simulink model "speedgoat_test_SN5659_R2021b"  (R2021b)
settings: Solver=FixedStepDiscrete  StartTime=0.0  StopTime=inf  RelTol=1e-3
PreLoadFcn:
  | Ts_IO107 = 0.001;
  | Ts_IO107 = 0.001;
  | Ts_IO133 = 0.001
  | 
  | Ts_IO204 = 0.001;
  | 
  | 
  | Ts_IO503 = 0.01;
  | 
  | ts_IO612 = 1e-3;
  | Ts_IO682 = 0.005;
  | Ts_IO941 = 0.01;
InitFcn:
  | Ts_IO107 = 0.001;
  | Ts_IO107 = 0.001;
  | Ts_IO133 = 0.001
  | 
  | Ts_IO204 = 0.001;
  | 
  | 
  | Ts_IO503 = 0.01;
  | 
  | ts_IO612 = 1e-3;
  | Ts_IO682 = 0.005;
  | Ts_IO941 = 0.01;
StopFcn:
  | if isfile(['sdi_view_',bdroot,'.mldatx'])
  |  Simulink.sdi.clearPreferences();
  |  Simulink.sdi.view();
  |  pause(3);
  |  Simulink.sdi.loadView(['sdi_view_',bdroot,]);
  | end
undefined symbols (not defined in the file): C, IO682, standard
libraries: speedgoatlib_IO682 x161, simulink x49, slrealtimeseriallib x16, canmsglib x12, speedgoatlib_serial x9, speedgoatlib_IO612 x9, speedgoatlib_IO133 x5, speedgoatlib_IO107 x4, speedgoatlib_IO204 x3, speedgoatlib_IO421 x3, speedgoatlib_PIL x1
(part 2 of 4)

== system speedgoat_test_SN5659_R2021b/IO682/Decode Channel 12 ==
  In1 : Inport
  Decode 1 : speedgoatlib_IO682/Decode v2   parMode=Standard  parLabel=100  parDataType=[1]  parResolution=[1024]  parSyncMask=hex2dec('0x0')  parSyncValue=hex2dec('0x0')  parCustomDataType=Raw  parDataLSB=9  parDataMSB=31  parBitPosition=[9, 31]  parScaleBNR=1  parExponent=8  parMantissa=14  parTimeTags=off  parHoldLastVal=on  parStatus=off
      settings: SourceProductName=Simulink Real-Time: Speedgoat I/O Blockset
  Decode 2 : speedgoatlib_IO682/Decode v2   parMode=Standard  parLabel=101  parDataType=[2]  parResolution=[.1]  parSyncMask=hex2dec('0x0')  parSyncValue=hex2dec('0x0')  parCustomDataType=Raw  parDataLSB=9  parDataMSB=31  parBitPosition=[9, 31]  parScaleBNR=1  parExponent=8  parMantissa=14  parTimeTags=off  parHoldLastVal=on  parStatus=off
      settings: SourceProductName=Simulink Real-Time: Speedgoat I/O Blockset
  Decode 3 : speedgoatlib_IO682/Decode v2   parMode=Standard  parLabel=102  parDataType=[1]  parResolution=[65536]  parSyncMask=hex2dec('0x0')  parSyncValue=hex2dec('0x0')  parCustomDataType=Raw  parDataLSB=9  parDataMSB=31  parBitPosition=[9, 31]  parScaleBNR=1  parExponent=8  parMantissa=14  parTimeTags=off  parHoldLastVal=on  parStatus=off
      settings: SourceProductName=Simulink Real-Time: Speedgoat I/O Blockset
  Decode 4 : speedgoatlib_IO682/Decode v2   parMode=Standard  parLabel=103  parDataType=[1]  parResolution=[1024]  parSyncMask=hex2dec('0x0')  parSyncValue=hex2dec('0x0')  parCustomDataType=Raw  parDataLSB=9  parDataMSB=31  parBitPosition=[9, 31]  parScaleBNR=1  parExponent=8  parMantissa=14  parTimeTags=off  parHoldLastVal=on  parStatus=off
      settings: SourceProductName=Simulink Real-Time: Speedgoat I/O Blockset
  Mux : Mux
  Out1 : Outport
  wires:
  Decode 1/1 -> Mux/1
  Decode 2/1 -> Mux/2
  Decode 4/1 -> Mux/4
  Decode 3/1 -> Mux/3
  Mux/1 -> Out1/1
  In1/1 -> Decode 4/1, Decode 3/1, Decode 2/1, Decode 1/1

== system speedgoat_test_SN5659_R2021b/IO682/Decode Channel 13 ==
  note: Because of the limited number of bits
      | that are encoded and sent by ARINC,
      | these values may differ from values
      | on the input side.
  In1 : Inport
  Decode 1 : speedgoatlib_IO682/Decode v2   parMode=Standard  parLabel=100  parDataType=[1]  parResolution=[1024]  parSyncMask=hex2dec('0x0')  parSyncValue=hex2dec('0x0')  parCustomDataType=Raw  parDataLSB=9  parDataMSB=31  parBitPosition=[9, 31]  parScaleBNR=1  parExponent=8  parMantissa=14  parTimeTags=off  parHoldLastVal=on  parStatus=off
      settings: SourceProductName=Simulink Real-Time: Speedgoat I/O Blockset
  Decode 3 : speedgoatlib_IO682/Decode v2   parMode=Standard  parLabel=102  parDataType=[1]  parResolution=[65536]  parSyncMask=hex2dec('0x0')  parSyncValue=hex2dec('0x0')  parCustomDataType=Raw  parDataLSB=9  parDataMSB=31  parBitPosition=[9, 31]  parScaleBNR=1  parExponent=8  parMantissa=14  parTimeTags=off  parHoldLastVal=on  parStatus=off
      settings: SourceProductName=Simulink Real-Time: Speedgoat I/O Blockset
  Decode 4 : speedgoatlib_IO682/Decode v2   parMode=Standard  parLabel=103  parDataType=[1]  parResolution=[1024]  parSyncMask=hex2dec('0x0')  parSyncValue=hex2dec('0x0')  parCustomDataType=Raw  parDataLSB=9  parDataMSB=31  parBitPosition=[9, 31]  parScaleBNR=1  parExponent=8  parMantissa=14  parTimeTags=off  parHoldLastVal=on  parStatus=off
      settings: SourceProductName=Simulink Real-Time: Speedgoat I/O Blockset
  Decode 5 : speedgoatlib_IO682/Decode v2   parMode=Standard  parLabel=101  parDataType=[2]  parResolution=[.1]  parSyncMask=hex2dec('0x0')  parSyncValue=hex2dec('0x0')  parCustomDataType=Raw  parDataLSB=9  parDataMSB=31  parBitPosition=[9, 31]  parScaleBNR=1  parExponent=8  parMantissa=14  parTimeTags=off  parHoldLastVal=on  parStatus=off
      settings: SourceProductName=Simulink Real-Time: Speedgoat I/O Blockset
  Mux : Mux
  Out1 : Outport
  wires:
  In1/1 -> Decode 3/1, Decode 4/1, Decode 5/1, Decode 1/1
  Mux/1 -> Out1/1
  Decode 5/1 -> Mux/2
  Decode 1/1 -> Mux/1
  Decode 3/1 -> Mux/3
  Decode 4/1 -> Mux/4

== system speedgoat_test_SN5659_R2021b/IO682/Decode Channel 14 ==
  In1 : Inport
  Decode 1 : speedgoatlib_IO682/Decode v2   parMode=Standard  parLabel=100  parDataType=[1]  parResolution=[1024]  parSyncMask=hex2dec('0x0')  parSyncValue=hex2dec('0x0')  parCustomDataType=Raw  parDataLSB=9  parDataMSB=31  parBitPosition=[9, 31]  parScaleBNR=1  parExponent=8  parMantissa=14  parTimeTags=off  parHoldLastVal=on  parStatus=off
      settings: SourceProductName=Simulink Real-Time: Speedgoat I/O Blockset
  Decode 2 : speedgoatlib_IO682/Decode v2   parMode=Standard  parLabel=101  parDataType=[2]  parResolution=[.1]  parSyncMask=hex2dec('0x0')  parSyncValue=hex2dec('0x0')  parCustomDataType=Raw  parDataLSB=9  parDataMSB=31  parBitPosition=[9, 31]  parScaleBNR=1  parExponent=8  parMantissa=14  parTimeTags=off  parHoldLastVal=on  parStatus=off
      settings: SourceProductName=Simulink Real-Time: Speedgoat I/O Blockset
  Decode 3 : speedgoatlib_IO682/Decode v2   parMode=Standard  parLabel=102  parDataType=[1]  parResolution=[65536]  parSyncMask=hex2dec('0x0')  parSyncValue=hex2dec('0x0')  parCustomDataType=Raw  parDataLSB=9  parDataMSB=31  parBitPosition=[9, 31]  parScaleBNR=1  parExponent=8  parMantissa=14  parTimeTags=off  parHoldLastVal=on  parStatus=off
      settings: SourceProductName=Simulink Real-Time: Speedgoat I/O Blockset
  Decode 4 : speedgoatlib_IO682/Decode v2   parMode=Standard  parLabel=103  parDataType=[1]  parResolution=[1024]  parSyncMask=hex2dec('0x0')  parSyncValue=hex2dec('0x0')  parCustomDataType=Raw  parDataLSB=9  parDataMSB=31  parBitPosition=[9, 31]  parScaleBNR=1  parExponent=8  parMantissa=14  parTimeTags=off  parHoldLastVal=on  parStatus=off
      settings: SourceProductName=Simulink Real-Time: Speedgoat I/O Blockset
  Mux : Mux
  Out1 : Outport
  wires:
  Decode 1/1 -> Mux/1
  In1/1 -> Decode 4/1, Decode 3/1, Decode 2/1, Decode 1/1
  Mux/1 -> Out1/1
  Decode 4/1 -> Mux/4
  Decode 3/1 -> Mux/3
  Decode 2/1 -> Mux/2

== system speedgoat_test_SN5659_R2021b/IO682/Decode Channel 15 ==
  In1 : Inport
  Decode 1 : speedgoatlib_IO682/Decode v2   parMode=Standard  parLabel=100  parDataType=[1]  parResolution=[1024]  parSyncMask=hex2dec('0x0')  parSyncValue=hex2dec('0x0')  parCustomDataType=Raw  parDataLSB=9  parDataMSB=31  parBitPosition=[9, 31]  parScaleBNR=1  parExponent=8  parMantissa=14  parTimeTags=off  parHoldLastVal=on  parStatus=off
      settings: SourceProductName=Simulink Real-Time: Speedgoat I/O Blockset
  Decode 2 : speedgoatlib_IO682/Decode v2   parMode=Standard  parLabel=101  parDataType=[2]  parResolution=[.1]  parSyncMask=hex2dec('0x0')  parSyncValue=hex2dec('0x0')  parCustomDataType=Raw  parDataLSB=9  parDataMSB=31  parBitPosition=[9, 31]  parScaleBNR=1  parExponent=8  parMantissa=14  parTimeTags=off  parHoldLastVal=on  parStatus=off
      settings: SourceProductName=Simulink Real-Time: Speedgoat I/O Blockset
  Decode 3 : speedgoatlib_IO682/Decode v2   parMode=Standard  parLabel=102  parDataType=[1]  parResolution=[65536]  parSyncMask=hex2dec('0x0')  parSyncValue=hex2dec('0x0')  parCustomDataType=Raw  parDataLSB=9  parDataMSB=31  parBitPosition=[9, 31]  parScaleBNR=1  parExponent=8  parMantissa=14  parTimeTags=off  parHoldLastVal=on  parStatus=off
      settings: SourceProductName=Simulink Real-Time: Speedgoat I/O Blockset
  Decode 4 : speedgoatlib_IO682/Decode v2   parMode=Standard  parLabel=103  parDataType=[1]  parResolution=[1024]  parSyncMask=hex2dec('0x0')  parSyncValue=hex2dec('0x0')  parCustomDataType=Raw  parDataLSB=9  parDataMSB=31  parBitPosition=[9, 31]  parScaleBNR=1  parExponent=8  parMantissa=14  parTimeTags=off  parHoldLastVal=on  parStatus=off
      settings: SourceProductName=Simulink Real-Time: Speedgoat I/O Blockset
  Mux : Mux
  Out1 : Outport
  wires:
  Decode 1/1 -> Mux/1
  Decode 2/1 -> Mux/2
  Decode 4/1 -> Mux/4
  Decode 3/1 -> Mux/3
  Mux/1 -> Out1/1
  In1/1 -> Decode 4/1, Decode 3/1, Decode 2/1, Decode 1/1

== system speedgoat_test_SN5659_R2021b/IO682/Decode Channel 16 ==
  In1 : Inport
  Decode 1 : speedgoatlib_IO682/Decode v2   parMode=Standard  parLabel=100  parDataType=[1]  parResolution=[1024]  parSyncMask=hex2dec('0x0')  parSyncValue=hex2dec('0x0')  parCustomDataType=Raw  parDataLSB=9  parDataMSB=31  parBitPosition=[9, 31]  parScaleBNR=1  parExponent=8  parMantissa=14  parTimeTags=off  parHoldLastVal=on  parStatus=off
      settings: SourceProductName=Simulink Real-Time: Speedgoat I/O Blockset
  Decode 2 : speedgoatlib_IO682/Decode v2   parMode=Standard  parLabel=101  parDataType=[2]  parResolution=[.1]  parSyncMask=hex2dec('0x0')  parSyncValue=hex2dec('0x0')  parCustomDataType=Raw  parDataLSB=9  parDataMSB=31  parBitPosition=[9, 31]  parScaleBNR=1  parExponent=8  parMantissa=14  parTimeTags=off  parHoldLastVal=on  parStatus=off
      settings: SourceProductName=Simulink Real-Time: Speedgoat I/O Blockset
  Decode 3 : speedgoatlib_IO682/Decode v2   parMode=Standard  parLabel=102  parDataType=[1]  parResolution=[65536]  parSyncMask=hex2dec('0x0')  parSyncValue=hex2dec('0x0')  parCustomDataType=Raw  parDataLSB=9  parDataMSB=31  parBitPosition=[9, 31]  parScaleBNR=1  parExponent=8  parMantissa=14  parTimeTags=off  parHoldLastVal=on  parStatus=off
      settings: SourceProductName=Simulink Real-Time: Speedgoat I/O Blockset
  Decode 4 : speedgoatlib_IO682/Decode v2   parMode=Standard  parLabel=103  parDataType=[1]  parResolution=[1024]  parSyncMask=hex2dec('0x0')  parSyncValue=hex2dec('0x0')  parCustomDataType=Raw  parDataLSB=9  parDataMSB=31  parBitPosition=[9, 31]  parScaleBNR=1  parExponent=8  parMantissa=14  parTimeTags=off  parHoldLastVal=on  parStatus=off
      settings: SourceProductName=Simulink Real-Time: Speedgoat I/O Blockset
  Mux : Mux
  Out1 : Outport
  wires:
  Decode 1/1 -> Mux/1
  Decode 2/1 -> Mux/2
  Decode 4/1 -> Mux/4
  Decode 3/1 -> Mux/3
  Mux/1 -> Out1/1
  In1/1 -> Decode 4/1, Decode 3/1, Decode 2/1, Decode 1/1

== system speedgoat_test_SN5659_R2021b/IO682/Decode Channel 2 ==
  In1 : Inport
  Decode 1 : speedgoatlib_IO682/Decode v2   parMode=Standard  parLabel=100  parDataType=[1]  parResolution=[1024]  parSyncMask=hex2dec('0x0')  parSyncValue=hex2dec('0x0')  parCustomDataType=Raw  parDataLSB=9  parDataMSB=31  parBitPosition=[9, 31]  parScaleBNR=1  parExponent=8  parMantissa=14  parTimeTags=off  parHoldLastVal=on  parStatus=off
      settings: SourceProductName=Simulink Real-Time: Speedgoat I/O Blockset
  Decode 2 : speedgoatlib_IO682/Decode v2   parMode=Standard  parLabel=101  parDataType=[2]  parResolution=[.1]  parSyncMask=hex2dec('0x0')  parSyncValue=hex2dec('0x0')  parCustomDataType=Raw  parDataLSB=9  parDataMSB=31  parBitPosition=[9, 31]  parScaleBNR=1  parExponent=8  parMantissa=14  parTimeTags=off  parHoldLastVal=on  parStatus=off
      settings: SourceProductName=Simulink Real-Time: Speedgoat I/O Blockset
  Decode 3 : speedgoatlib_IO682/Decode v2   parMode=Standard  parLabel=102  parDataType=[1]  parResolution=[65536]  parSyncMask=hex2dec('0x0')  parSyncValue=hex2dec('0x0')  parCustomDataType=Raw  parDataLSB=9  parDataMSB=31  parBitPosition=[9, 31]  parScaleBNR=1  parExponent=8  parMantissa=14  parTimeTags=off  parHoldLastVal=on  parStatus=off
      settings: SourceProductName=Simulink Real-Time: Speedgoat I/O Blockset
  Decode 4 : speedgoatlib_IO682/Decode v2   parMode=Standard  parLabel=103  parDataType=[1]  parResolution=[1024]  parSyncMask=hex2dec('0x0')  parSyncValue=hex2dec('0x0')  parCustomDataType=Raw  parDataLSB=9  parDataMSB=31  parBitPosition=[9, 31]  parScaleBNR=1  parExponent=8  parMantissa=14  parTimeTags=off  parHoldLastVal=on  parStatus=off
      settings: SourceProductName=Simulink Real-Time: Speedgoat I/O Blockset
  Mux : Mux
  Out1 : Outport
  wires:
  Decode 1/1 -> Mux/1
  In1/1 -> Decode 4/1, Decode 3/1, Decode 2/1, Decode 1/1
  Mux/1 -> Out1/1
  Decode 4/1 -> Mux/4
  Decode 3/1 -> Mux/3
  Decode 2/1 -> Mux/2

== system speedgoat_test_SN5659_R2021b/IO682/Decode Channel 3 ==
  In1 : Inport
  Decode 1 : speedgoatlib_IO682/Decode v2   parMode=Standard  parLabel=100  parDataType=[1]  parResolution=[1024]  parSyncMask=hex2dec('0x0')  parSyncValue=hex2dec('0x0')  parCustomDataType=Raw  parDataLSB=9  parDataMSB=31  parBitPosition=[9, 31]  parScaleBNR=1  parExponent=8  parMantissa=14  parTimeTags=off  parHoldLastVal=on  parStatus=off
      settings: SourceProductName=Simulink Real-Time: Speedgoat I/O Blockset
  Decode 2 : speedgoatlib_IO682/Decode v2   parMode=Standard  parLabel=101  parDataType=[2]  parResolution=[.1]  parSyncMask=hex2dec('0x0')  parSyncValue=hex2dec('0x0')  parCustomDataType=Raw  parDataLSB=9  parDataMSB=31  parBitPosition=[9, 31]  parScaleBNR=1  parExponent=8  parMantissa=14  parTimeTags=off  parHoldLastVal=on  parStatus=off
      settings: SourceProductName=Simulink Real-Time: Speedgoat I/O Blockset
  Decode 3 : speedgoatlib_IO682/Decode v2   parMode=Standard  parLabel=102  parDataType=[1]  parResolution=[65536]  parSyncMask=hex2dec('0x0')  parSyncValue=hex2dec('0x0')  parCustomDataType=Raw  parDataLSB=9  parDataMSB=31  parBitPosition=[9, 31]  parScaleBNR=1  parExponent=8  parMantissa=14  parTimeTags=off  parHoldLastVal=on  parStatus=off
      settings: SourceProductName=Simulink Real-Time: Speedgoat I/O Blockset
  Decode 4 : speedgoatlib_IO682/Decode v2   parMode=Standard  parLabel=103  parDataType=[1]  parResolution=[1024]  parSyncMask=hex2dec('0x0')  parSyncValue=hex2dec('0x0')  parCustomDataType=Raw  parDataLSB=9  parDataMSB=31  parBitPosition=[9, 31]  parScaleBNR=1  parExponent=8  parMantissa=14  parTimeTags=off  parHoldLastVal=on  parStatus=off
      settings: SourceProductName=Simulink Real-Time: Speedgoat I/O Blockset
  Mux : Mux
  Out1 : Outport
  wires:
  Decode 1/1 -> Mux/1
  Decode 2/1 -> Mux/2
  Decode 4/1 -> Mux/4
  Decode 3/1 -> Mux/3
  Mux/1 -> Out1/1
  In1/1 -> Decode 4/1, Decode 3/1, Decode 2/1, Decode 1/1

== system speedgoat_test_SN5659_R2021b/IO682/Decode Channel 4 ==
  In1 : Inport
  Decode 1 : speedgoatlib_IO682/Decode v2   parMode=Standard  parLabel=100  parDataType=[1]  parResolution=[1024]  parSyncMask=hex2dec('0x0')  parSyncValue=hex2dec('0x0')  parCustomDataType=Raw  parDataLSB=9  parDataMSB=31  parBitPosition=[9, 31]  parScaleBNR=1  parExponent=8  parMantissa=14  parTimeTags=off  parHoldLastVal=on  parStatus=off
      settings: SourceProductName=Simulink Real-Time: Speedgoat I/O Blockset
  Decode 2 : speedgoatlib_IO682/Decode v2   parMode=Standard  parLabel=101  parDataType=[2]  parResolution=[.1]  parSyncMask=hex2dec('0x0')  parSyncValue=hex2dec('0x0')  parCustomDataType=Raw  parDataLSB=9  parDataMSB=31  parBitPosition=[9, 31]  parScaleBNR=1  parExponent=8  parMantissa=14  parTimeTags=off  parHoldLastVal=on  parStatus=off
      settings: SourceProductName=Simulink Real-Time: Speedgoat I/O Blockset
  Decode 3 : speedgoatlib_IO682/Decode v2   parMode=Standard  parLabel=102  parDataType=[1]  parResolution=[65536]  parSyncMask=hex2dec('0x0')  parSyncValue=hex2dec('0x0')  parCustomDataType=Raw  parDataLSB=9  parDataMSB=31  parBitPosition=[9, 31]  parScaleBNR=1  parExponent=8  parMantissa=14  parTimeTags=off  parHoldLastVal=on  parStatus=off
      settings: SourceProductName=Simulink Real-Time: Speedgoat I/O Blockset
  Decode 4 : speedgoatlib_IO682/Decode v2   parMode=Standard  parLabel=103  parDataType=[1]  parResolution=[1024]  parSyncMask=hex2dec('0x0')  parSyncValue=hex2dec('0x0')  parCustomDataType=Raw  parDataLSB=9  parDataMSB=31  parBitPosition=[9, 31]  parScaleBNR=1  parExponent=8  parMantissa=14  parTimeTags=off  parHoldLastVal=on  parStatus=off
      settings: SourceProductName=Simulink Real-Time: Speedgoat I/O Blockset
  Mux : Mux
  Out1 : Outport
  wires:
  Decode 1/1 -> Mux/1
  Decode 2/1 -> Mux/2
  Decode 4/1 -> Mux/4
  Decode 3/1 -> Mux/3
  Mux/1 -> Out1/1
  In1/1 -> Decode 4/1, Decode 3/1, Decode 2/1, Decode 1/1

== system speedgoat_test_SN5659_R2021b/IO682/Decode Channel 5 ==
  note: Because of the limited number of bits
      | that are encoded and sent by ARINC,
      | these values may differ from values
      | on the input side.
  In1 : Inport
  Decode 1 : speedgoatlib_IO682/Decode v2   parMode=Standard  parLabel=100  parDataType=[1]  parResolution=[1024]  parSyncMask=hex2dec('0x0')  parSyncValue=hex2dec('0x0')  parCustomDataType=Raw  parDataLSB=9  parDataMSB=31  parBitPosition=[9, 31]  parScaleBNR=1  parExponent=8  parMantissa=14  parTimeTags=off  parHoldLastVal=on  parStatus=off
      settings: SourceProductName=Simulink Real-Time: Speedgoat I/O Blockset
  Decode 3 : speedgoatlib_IO682/Decode v2   parMode=Standard  parLabel=102  parDataType=[1]  parResolution=[65536]  parSyncMask=hex2dec('0x0')  parSyncValue=hex2dec('0x0')  parCustomDataType=Raw  parDataLSB=9  parDataMSB=31  parBitPosition=[9, 31]  parScaleBNR=1  parExponent=8  parMantissa=14  parTimeTags=off  parHoldLastVal=on  parStatus=off
      settings: SourceProductName=Simulink Real-Time: Speedgoat I/O Blockset
  Decode 4 : speedgoatlib_IO682/Decode v2   parMode=Standard  parLabel=103  parDataType=[1]  parResolution=[1024]  parSyncMask=hex2dec('0x0')  parSyncValue=hex2dec('0x0')  parCustomDataType=Raw  parDataLSB=9  parDataMSB=31  parBitPosition=[9, 31]  parScaleBNR=1  parExponent=8  parMantissa=14  parTimeTags=off  parHoldLastVal=on  parStatus=off
      settings: SourceProductName=Simulink Real-Time: Speedgoat I/O Blockset
  Decode 5 : speedgoatlib_IO682/Decode v2   parMode=Standard  parLabel=101  parDataType=[2]  parResolution=[.1]  parSyncMask=hex2dec('0x0')  parSyncValue=hex2dec('0x0')  parCustomDataType=Raw  parDataLSB=9  parDataMSB=31  parBitPosition=[9, 31]  parScaleBNR=1  parExponent=8  parMantissa=14  parTimeTags=off  parHoldLastVal=on  parStatus=off
      settings: SourceProductName=Simulink Real-Time: Speedgoat I/O Blockset
  Mux : Mux
  Out1 : Outport
  wires:
  In1/1 -> Decode 3/1, Decode 4/1, Decode 5/1, Decode 1/1
  Mux/1 -> Out1/1
  Decode 5/1 -> Mux/2
  Decode 1/1 -> Mux/1
  Decode 3/1 -> Mux/3
  Decode 4/1 -> Mux/4

== system speedgoat_test_SN5659_R2021b/IO682/Decode Channel 6 ==
  In1 : Inport
  Decode 1 : speedgoatlib_IO682/Decode v2   parMode=Standard  parLabel=100  parDataType=[1]  parResolution=[1024]  parSyncMask=hex2dec('0x0')  parSyncValue=hex2dec('0x0')  parCustomDataType=Raw  parDataLSB=9  parDataMSB=31  parBitPosition=[9, 31]  parScaleBNR=1  parExponent=8  parMantissa=14  parTimeTags=off  parHoldLastVal=on  parStatus=off
      settings: SourceProductName=Simulink Real-Time: Speedgoat I/O Blockset
  Decode 2 : speedgoatlib_IO682/Decode v2   parMode=Standard  parLabel=101  parDataType=[2]  parResolution=[.1]  parSyncMask=hex2dec('0x0')  parSyncValue=hex2dec('0x0')  parCustomDataType=Raw  parDataLSB=9  parDataMSB=31  parBitPosition=[9, 31]  parScaleBNR=1  parExponent=8  parMantissa=14  parTimeTags=off  parHoldLastVal=on  parStatus=off
      settings: SourceProductName=Simulink Real-Time: Speedgoat I/O Blockset
  Decode 3 : speedgoatlib_IO682/Decode v2   parMode=Standard  parLabel=102  parDataType=[1]  parResolution=[65536]  parSyncMask=hex2dec('0x0')  parSyncValue=hex2dec('0x0')  parCustomDataType=Raw  parDataLSB=9  parDataMSB=31  parBitPosition=[9, 31]  parScaleBNR=1  parExponent=8  parMantissa=14  parTimeTags=off  parHoldLastVal=on  parStatus=off
      settings: SourceProductName=Simulink Real-Time: Speedgoat I/O Blockset
  Decode 4 : speedgoatlib_IO682/Decode v2   parMode=Standard  parLabel=103  parDataType=[1]  parResolution=[1024]  parSyncMask=hex2dec('0x0')  parSyncValue=hex2dec('0x0')  parCustomDataType=Raw  parDataLSB=9  parDataMSB=31  parBitPosition=[9, 31]  parScaleBNR=1  parExponent=8  parMantissa=14  parTimeTags=off  parHoldLastVal=on  parStatus=off
      settings: SourceProductName=Simulink Real-Time: Speedgoat I/O Blockset
  Mux : Mux
  Out1 : Outport
  wires:
  Decode 1/1 -> Mux/1
  In1/1 -> Decode 4/1, Decode 3/1, Decode 2/1, Decode 1/1
  Mux/1 -> Out1/1
  Decode 4/1 -> Mux/4
  Decode 3/1 -> Mux/3
  Decode 2/1 -> Mux/2

== system speedgoat_test_SN5659_R2021b/IO682/Decode Channel 7 ==
  In1 : Inport
  Decode 1 : speedgoatlib_IO682/Decode v2   parMode=Standard  parLabel=100  parDataType=[1]  parResolution=[1024]  parSyncMask=hex2dec('0x0')  parSyncValue=hex2dec('0x0')  parCustomDataType=Raw  parDataLSB=9  parDataMSB=31  parBitPosition=[9, 31]  parScaleBNR=1  parExponent=8  parMantissa=14  parTimeTags=off  parHoldLastVal=on  parStatus=off
      settings: SourceProductName=Simulink Real-Time: Speedgoat I/O Blockset
  Decode 2 : speedgoatlib_IO682/Decode v2   parMode=Standard  parLabel=101  parDataType=[2]  parResolution=[.1]  parSyncMask=hex2dec('0x0')  parSyncValue=hex2dec('0x0')  parCustomDataType=Raw  parDataLSB=9  parDataMSB=31  parBitPosition=[9, 31]  parScaleBNR=1  parExponent=8  parMantissa=14  parTimeTags=off  parHoldLastVal=on  parStatus=off
      settings: SourceProductName=Simulink Real-Time: Speedgoat I/O Blockset
  Decode 3 : speedgoatlib_IO682/Decode v2   parMode=Standard  parLabel=102  parDataType=[1]  parResolution=[65536]  parSyncMask=hex2dec('0x0')  parSyncValue=hex2dec('0x0')  parCustomDataType=Raw  parDataLSB=9  parDataMSB=31  parBitPosition=[9, 31]  parScaleBNR=1  parExponent=8  parMantissa=14  parTimeTags=off  parHoldLastVal=on  parStatus=off
      settings: SourceProductName=Simulink Real-Time: Speedgoat I/O Blockset
  Decode 4 : speedgoatlib_IO682/Decode v2   parMode=Standard  parLabel=103  parDataType=[1]  parResolution=[1024]  parSyncMask=hex2dec('0x0')  parSyncValue=hex2dec('0x0')  parCustomDataType=Raw  parDataLSB=9  parDataMSB=31  parBitPosition=[9, 31]  parScaleBNR=1  parExponent=8  parMantissa=14  parTimeTags=off  parHoldLastVal=on  parStatus=off
      settings: SourceProductName=Simulink Real-Time: Speedgoat I/O Blockset
  Mux : Mux
  Out1 : Outport
  wires:
  Decode 1/1 -> Mux/1
  Decode 2/1 -> Mux/2
  Decode 4/1 -> Mux/4
  Decode 3/1 -> Mux/3
  Mux/1 -> Out1/1
  In1/1 -> Decode 4/1, Decode 3/1, Decode 2/1, Decode 1/1

== system speedgoat_test_SN5659_R2021b/IO682/Decode Channel 8 ==
  In1 : Inport
  Decode 1 : speedgoatlib_IO682/Decode v2   parMode=Standard  parLabel=100  parDataType=[1]  parResolution=[1024]  parSyncMask=hex2dec('0x0')  parSyncValue=hex2dec('0x0')  parCustomDataType=Raw  parDataLSB=9  parDataMSB=31  parBitPosition=[9, 31]  parScaleBNR=1  parExponent=8  parMantissa=14  parTimeTags=off  parHoldLastVal=on  parStatus=off
      settings: SourceProductName=Simulink Real-Time: Speedgoat I/O Blockset
  Decode 2 : speedgoatlib_IO682/Decode v2   parMode=Standard  parLabel=101  parDataType=[2]  parResolution=[.1]  parSyncMask=hex2dec('0x0')  parSyncValue=hex2dec('0x0')  parCustomDataType=Raw  parDataLSB=9  parDataMSB=31  parBitPosition=[9, 31]  parScaleBNR=1  parExponent=8  parMantissa=14  parTimeTags=off  parHoldLastVal=on  parStatus=off
      settings: SourceProductName=Simulink Real-Time: Speedgoat I/O Blockset
  Decode 3 : speedgoatlib_IO682/Decode v2   parMode=Standard  parLabel=102  parDataType=[1]  parResolution=[65536]  parSyncMask=hex2dec('0x0')  parSyncValue=hex2dec('0x0')  parCustomDataType=Raw  parDataLSB=9  parDataMSB=31  parBitPosition=[9, 31]  parScaleBNR=1  parExponent=8  parMantissa=14  parTimeTags=off  parHoldLastVal=on  parStatus=off
      settings: SourceProductName=Simulink Real-Time: Speedgoat I/O Blockset
  Decode 4 : speedgoatlib_IO682/Decode v2   parMode=Standard  parLabel=103  parDataType=[1]  parResolution=[1024]  parSyncMask=hex2dec('0x0')  parSyncValue=hex2dec('0x0')  parCustomDataType=Raw  parDataLSB=9  parDataMSB=31  parBitPosition=[9, 31]  parScaleBNR=1  parExponent=8  parMantissa=14  parTimeTags=off  parHoldLastVal=on  parStatus=off
      settings: SourceProductName=Simulink Real-Time: Speedgoat I/O Blockset
  Mux : Mux
  Out1 : Outport
  wires:
  Decode 1/1 -> Mux/1
  Decode 2/1 -> Mux/2
  Decode 4/1 -> Mux/4
  Decode 3/1 -> Mux/3
  Mux/1 -> Out1/1
  In1/1 -> Decode 4/1, Decode 3/1, Decode 2/1, Decode 1/1

== system speedgoat_test_SN5659_R2021b/IO682/Decode Channel 9 ==
  note: Because of the limited number of bits
      | that are encoded and sent by ARINC,
      | these values may differ from values
      | on the input side.
  In1 : Inport
  Decode 1 : speedgoatlib_IO682/Decode v2   parMode=Standard  parLabel=100  parDataType=[1]  parResolution=[1024]  parSyncMask=hex2dec('0x0')  parSyncValue=hex2dec('0x0')  parCustomDataType=Raw  parDataLSB=9  parDataMSB=31  parBitPosition=[9, 31]  parScaleBNR=1  parExponent=8  parMantissa=14  parTimeTags=off  parHoldLastVal=on  parStatus=off
      settings: SourceProductName=Simulink Real-Time: Speedgoat I/O Blockset
  Decode 3 : speedgoatlib_IO682/Decode v2   parMode=Standard  parLabel=102  parDataType=[1]  parResolution=[65536]  parSyncMask=hex2dec('0x0')  parSyncValue=hex2dec('0x0')  parCustomDataType=Raw  parDataLSB=9  parDataMSB=31  parBitPosition=[9, 31]  parScaleBNR=1  parExponent=8  parMantissa=14  parTimeTags=off  parHoldLastVal=on  parStatus=off
      settings: SourceProductName=Simulink Real-Time: Speedgoat I/O Blockset
  Decode 4 : speedgoatlib_IO682/Decode v2   parMode=Standard  parLabel=103  parDataType=[1]  parResolution=[1024]  parSyncMask=hex2dec('0x0')  parSyncValue=hex2dec('0x0')  parCustomDataType=Raw  parDataLSB=9  parDataMSB=31  parBitPosition=[9, 31]  parScaleBNR=1  parExponent=8  parMantissa=14  parTimeTags=off  parHoldLastVal=on  parStatus=off
      settings: SourceProductName=Simulink Real-Time: Speedgoat I/O Blockset
  Decode 5 : speedgoatlib_IO682/Decode v2   parMode=Standard  parLabel=101  parDataType=[2]  parResolution=[.1]  parSyncMask=hex2dec('0x0')  parSyncValue=hex2dec('0x0')  parCustomDataType=Raw  parDataLSB=9  parDataMSB=31  parBitPosition=[9, 31]  parScaleBNR=1  parExponent=8  parMantissa=14  parTimeTags=off  parHoldLastVal=on  parStatus=off
      settings: SourceProductName=Simulink Real-Time: Speedgoat I/O Blockset
  Mux : Mux
  Out1 : Outport
  wires:
  In1/1 -> Decode 3/1, Decode 4/1, Decode 5/1, Decode 1/1
  Mux/1 -> Out1/1
  Decode 5/1 -> Mux/2
  Decode 1/1 -> Mux/1
  Decode 3/1 -> Mux/3
  Decode 4/1 -> Mux/4

== system speedgoat_test_SN5659_R2021b/IO682/Encode Channel 1 ==
  note: Encode block definitions:
      | 1. Label 100, BNR, Scale 1024, 10 bits, SDI 2, SSM 3
      | 2. Label 101, BCD, Resolution 0.1, SDI 2, SSM from sign of input
      | 3. Label 102, BNR, Scale 65536, 16 bits, SDI 2, SSM 3
      | 4. Label 103, RAW, Resolution/Scale, SDI and SSM aren't taken
      |         from the Encode block mask, but leave placeholders in the arrays.
      |         These values are inserted into the RAW value in the Prepare
      |         RAW value subsystem.  Label is also inserted manually.
  Constant : Constant  Value=50.159  SampleTime=Ts_IO682
  Counter Limited : simulink/Sources/Counter Limited  uplimit=100  tsamp=Ts_IO682
  Data Type Conversion : DataTypeConversion
  Encode 1 : speedgoatlib_IO682/Encode v2   parMode=Message Sequence  parLabel=100  parDataType=[1]  parResolution=[1024]  parBits=[10]  parSdi=[2]  parSsm=[3]  parCustomDataType=Raw  parDataLSB=9  parDataMSB=31  parBitPosition=[9, 31]  parScaleBNR=1  parExponent=8  parMantissa=14  parEnSSM=off
      settings: SourceProductName=Simulink Real-Time: Speedgoat I/O Blockset
  Encode 2 : speedgoatlib_IO682/Encode v2   parMode=Message Sequence  parLabel=103  parDataType=[0]  parResolution=[1024]  parBits=[0]  parSdi=[0]  parSsm=[0]  parCustomDataType=Raw  parDataLSB=9  parDataMSB=31  parBitPosition=[9, 31]  parScaleBNR=1  parExponent=8  parMantissa=14  parEnSSM=off
      settings: SourceProductName=Simulink Real-Time: Speedgoat I/O Blockset
  Encode 3 : speedgoatlib_IO682/Encode v2   parMode=Message Sequence  parLabel=102  parDataType=[1]  parResolution=[65536]  parBits=[16]  parSdi=[2]  parSsm=[3]  parCustomDataType=Raw  parDataLSB=9  parDataMSB=31  parBitPosition=[9, 31]  parScaleBNR=1  parExponent=8  parMantissa=14  parEnSSM=off
      settings: SourceProductName=Simulink Real-Time: Speedgoat I/O Blockset
  Encode 5 : speedgoatlib_IO682/Encode v2   parMode=Message Sequence  parLabel=101  parDataType=[2]  parResolution=[.1]  parBits=[0]  parSdi=[2]  parSsm=[0]  parCustomDataType=Raw  parDataLSB=9  parDataMSB=31  parBitPosition=[9, 31]  parScaleBNR=1  parExponent=8  parMantissa=14  parEnSSM=off
      settings: SourceProductName=Simulink Real-Time: Speedgoat I/O Blockset
  Mux : Mux
  Prepare RAW value : Subsystem
  Random number : RandomNumber  Mean=50  Variance=10  SampleTime=Ts_IO682
  Sine wave : Sin  Amplitude=10000  Bias=11000  Frequency=2*pi*0.01  SampleTime=Ts_IO682
  Out1 : Outport
  wires:
  Mux/1 -> Out1/1
  Sine wave/1 -> Encode 3/1
  Encode 2/1 -> Mux/4
  Encode 3/1 -> Mux/3
  Encode 5/1 -> Mux/2
  Random number/1 -> Encode 1/1
  Encode 1/1 -> Mux/1
  Counter Limited/1 -> Data Type Conversion/1
  Prepare RAW value/1(Out1) -> Encode 2/1
  Constant/1 -> Prepare RAW value/1(In1)
  Data Type Conversion/1 -> Encode 5/1

== system speedgoat_test_SN5659_R2021b/IO682/Encode Channel 10 ==
  Constant : Constant  Value=500.159  SampleTime=Ts_IO682
  Counter Limited : simulink/Sources/Counter Limited  uplimit=1000  tsamp=Ts_IO682
  Data Type Conversion : DataTypeConversion
  Encode 1 : speedgoatlib_IO682/Encode v2   parMode=Message Sequence  parLabel=100  parDataType=[1]  parResolution=[1024]  parBits=[10]  parSdi=[2]  parSsm=[3]  parCustomDataType=Raw  parDataLSB=9  parDataMSB=31  parBitPosition=[9, 31]  parScaleBNR=1  parExponent=8  parMantissa=14  parEnSSM=off
      settings: SourceProductName=Simulink Real-Time: Speedgoat I/O Blockset
  Encode 2 : speedgoatlib_IO682/Encode v2   parMode=Message Sequence  parLabel=101  parDataType=[2]  parResolution=[.1]  parBits=[0]  parSdi=[2]  parSsm=[0]  parCustomDataType=Raw  parDataLSB=9  parDataMSB=31  parBitPosition=[9, 31]  parScaleBNR=1  parExponent=8  parMantissa=14  parEnSSM=off
      settings: SourceProductName=Simulink Real-Time: Speedgoat I/O Blockset
  Encode 3 : speedgoatlib_IO682/Encode v2   parMode=Message Sequence  parLabel=102  parDataType=[1]  parResolution=[65536]  parBits=[16]  parSdi=[2]  parSsm=[3]  parCustomDataType=Raw  parDataLSB=9  parDataMSB=31  parBitPosition=[9, 31]  parScaleBNR=1  parExponent=8  parMantissa=14  parEnSSM=off
      settings: SourceProductName=Simulink Real-Time: Speedgoat I/O Blockset
  Encode 4 : speedgoatlib_IO682/Encode v2   parMode=Message Sequence  parLabel=103  parDataType=[0]  parResolution=[1]  parBits=[0]  parSdi=[0]  parSsm=[0]  parCustomDataType=Raw  parDataLSB=9  parDataMSB=31  parBitPosition=[9, 31]  parScaleBNR=1  parExponent=8  parMantissa=14  parEnSSM=off
      settings: SourceProductName=Simulink Real-Time: Speedgoat I/O Blockset
  Mux1 : Mux
  Prepare RAW value : Subsystem
  Random number : RandomNumber  Mean=500  Variance=10  SampleTime=Ts_IO682
  Sine wave : Sin  Amplitude=10000  Bias=20000  Frequency=2*pi*0.01  SampleTime=Ts_IO682
  Out1 : Outport
  wires:
  Encode 2/1 -> Mux1/2
  Prepare RAW value/1(Out1) -> Encode 4/1
  Encode 3/1 -> Mux1/3
  Encode 1/1 -> Mux1/1
  Constant/1 -> Prepare RAW value/1(In1)
  Sine wave/1 -> Encode 3/1
  Random number/1 -> Encode 1/1
  Mux1/1 -> Out1/1
  Counter Limited/1 -> Data Type Conversion/1
  Encode 4/1 -> Mux1/4
  Data Type Conversion/1 -> Encode 2/1

== system speedgoat_test_SN5659_R2021b/IO682/Encode Channel 11 ==
  Constant : Constant  Value=550.159  SampleTime=Ts_IO682
  Counter Limited : simulink/Sources/Counter Limited  uplimit=1100  tsamp=Ts_IO682
  Data Type Conversion : DataTypeConversion
  Encode 1 : speedgoatlib_IO682/Encode v2   parMode=Message Sequence  parLabel=100  parDataType=[1]  parResolution=[1024]  parBits=[10]  parSdi=[2]  parSsm=[3]  parCustomDataType=Raw  parDataLSB=9  parDataMSB=31  parBitPosition=[9, 31]  parScaleBNR=1  parExponent=8  parMantissa=14  parEnSSM=off
      settings: SourceProductName=Simulink Real-Time: Speedgoat I/O Blockset
  Encode 2 : speedgoatlib_IO682/Encode v2   parMode=Message Sequence  parLabel=101  parDataType=[2]  parResolution=[.1]  parBits=[0]  parSdi=[2]  parSsm=[0]  parCustomDataType=Raw  parDataLSB=9  parDataMSB=31  parBitPosition=[9, 31]  parScaleBNR=1  parExponent=8  parMantissa=14  parEnSSM=off
      settings: SourceProductName=Simulink Real-Time: Speedgoat I/O Blockset
  Encode 3 : speedgoatlib_IO682/Encode v2   parMode=Message Sequence  parLabel=102  parDataType=[1]  parResolution=[65536]  parBits=[16]  parSdi=[2]  parSsm=[3]  parCustomDataType=Raw  parDataLSB=9  parDataMSB=31  parBitPosition=[9, 31]  parScaleBNR=1  parExponent=8  parMantissa=14  parEnSSM=off
      settings: SourceProductName=Simulink Real-Time: Speedgoat I/O Blockset
  Encode 4 : speedgoatlib_IO682/Encode v2   parMode=Message Sequence  parLabel=103  parDataType=[0]  parResolution=[1]  parBits=[0]  parSdi=[0]  parSsm=[0]  parCustomDataType=Raw  parDataLSB=9  parDataMSB=31  parBitPosition=[9, 31]  parScaleBNR=1  parExponent=8  parMantissa=14  parEnSSM=off
      settings: SourceProductName=Simulink Real-Time: Speedgoat I/O Blockset
  Mux1 : Mux
  Prepare RAW value : Subsystem
  Random number : RandomNumber  Mean=550  Variance=10  SampleTime=Ts_IO682
  Sine wave : Sin  Amplitude=10000  Bias=21000  Frequency=2*pi*0.01  SampleTime=Ts_IO682
  Out1 : Outport
  wires:
  Encode 4/1 -> Mux1/4
  Mux1/1 -> Out1/1
  Counter Limited/1 -> Data Type Conversion/1
  Sine wave/1 -> Encode 3/1
  Encode 3/1 -> Mux1/3
  Encode 1/1 -> Mux1/1
  Random number/1 -> Encode 1/1
  Encode 2/1 -> Mux1/2
  Prepare RAW value/1(Out1) -> Encode 4/1
  Constant/1 -> Prepare RAW value/1(In1)
  Data Type Conversion/1 -> Encode 2/1

== system speedgoat_test_SN5659_R2021b/IO682/Encode Channel 12 ==
  Constant : Constant  Value=600.159  SampleTime=Ts_IO682
  Counter Limited : simulink/Sources/Counter Limited  uplimit=1200  tsamp=Ts_IO682
  Data Type Conversion : DataTypeConversion
  Encode 1 : speedgoatlib_IO682/Encode v2   parMode=Message Sequence  parLabel=100  parDataType=[1]  parResolution=[1024]  parBits=[10]  parSdi=[2]  parSsm=[3]  parCustomDataType=Raw  parDataLSB=9  parDataMSB=31  parBitPosition=[9, 31]  parScaleBNR=1  parExponent=8  parMantissa=14  parEnSSM=off
      settings: SourceProductName=Simulink Real-Time: Speedgoat I/O Blockset
  Encode 2 : speedgoatlib_IO682/Encode v2   parMode=Message Sequence  parLabel=101  parDataType=[2]  parResolution=[.1]  parBits=[0]  parSdi=[2]  parSsm=[0]  parCustomDataType=Raw  parDataLSB=9  parDataMSB=31  parBitPosition=[9, 31]  parScaleBNR=1  parExponent=8  parMantissa=14  parEnSSM=off
      settings: SourceProductName=Simulink Real-Time: Speedgoat I/O Blockset
  Encode 3 : speedgoatlib_IO682/Encode v2   parMode=Message Sequence  parLabel=102  parDataType=[1]  parResolution=[65536]  parBits=[16]  parSdi=[2]  parSsm=[3]  parCustomDataType=Raw  parDataLSB=9  parDataMSB=31  parBitPosition=[9, 31]  parScaleBNR=1  parExponent=8  parMantissa=14  parEnSSM=off
      settings: SourceProductName=Simulink Real-Time: Speedgoat I/O Blockset
  Encode 4 : speedgoatlib_IO682/Encode v2   parMode=Message Sequence  parLabel=103  parDataType=[0]  parResolution=[1]  parBits=[0]  parSdi=[0]  parSsm=[0]  parCustomDataType=Raw  parDataLSB=9  parDataMSB=31  parBitPosition=[9, 31]  parScaleBNR=1  parExponent=8  parMantissa=14  parEnSSM=off
      settings: SourceProductName=Simulink Real-Time: Speedgoat I/O Blockset
  Mux1 : Mux
  Prepare RAW value : Subsystem
  Random number : RandomNumber  Mean=600  Variance=10  SampleTime=Ts_IO682
  Sine wave : Sin  Amplitude=10000  Bias=22000  Frequency=2*pi*0.01  SampleTime=Ts_IO682
  Out1 : Outport
  wires:
  Encode 4/1 -> Mux1/4
  Mux1/1 -> Out1/1
  Counter Limited/1 -> Data Type Conversion/1
  Sine wave/1 -> Encode 3/1
  Encode 3/1 -> Mux1/3
  Encode 1/1 -> Mux1/1
  Random number/1 -> Encode 1/1
  Encode 2/1 -> Mux1/2
  Prepare RAW value/1(Out1) -> Encode 4/1
  Constant/1 -> Prepare RAW value/1(In1)
  Data Type Conversion/1 -> Encode 2/1

== system speedgoat_test_SN5659_R2021b/IO682/Encode Channel 13 ==
  note: Encode block definitions:
      | 1. Label 100, BNR, Scale 1024, 10 bits, SDI 2, SSM 3
      | 2. Label 101, BCD, Resolution 0.1, SDI 2, SSM from sign of input
      | 3. Label 102, BNR, Scale 65536, 16 bits, SDI 2, SSM 3
      | 4. Label 103, RAW, Resolution/Scale, SDI and SSM aren't taken
      |         from the Encode block mask, but leave placeholders in the arrays.
      |         These values are inserted into the RAW value in the Prepare
      |         RAW value subsystem.  Label is also inserted manually.
  Constant : Constant  Value=650.159  SampleTime=Ts_IO682
  Counter Limited : simulink/Sources/Counter Limited  uplimit=1300  tsamp=Ts_IO682
  Data Type Conversion : DataTypeConversion
  Encode 1 : speedgoatlib_IO682/Encode v2   parMode=Message Sequence  parLabel=100  parDataType=[1]  parResolution=[1024]  parBits=[10]  parSdi=[2]  parSsm=[3]  parCustomDataType=Raw  parDataLSB=9  parDataMSB=31  parBitPosition=[9, 31]  parScaleBNR=1  parExponent=8  parMantissa=14  parEnSSM=off
      settings: SourceProductName=Simulink Real-Time: Speedgoat I/O Blockset
  Encode 2 : speedgoatlib_IO682/Encode v2   parMode=Message Sequence  parLabel=103  parDataType=[0]  parResolution=[1024]  parBits=[0]  parSdi=[0]  parSsm=[0]  parCustomDataType=Raw  parDataLSB=9  parDataMSB=31  parBitPosition=[9, 31]  parScaleBNR=1  parExponent=8  parMantissa=14  parEnSSM=off
      settings: SourceProductName=Simulink Real-Time: Speedgoat I/O Blockset
  Encode 3 : speedgoatlib_IO682/Encode v2   parMode=Message Sequence  parLabel=102  parDataType=[1]  parResolution=[65536]  parBits=[16]  parSdi=[2]  parSsm=[3]  parCustomDataType=Raw  parDataLSB=9  parDataMSB=31  parBitPosition=[9, 31]  parScaleBNR=1  parExponent=8  parMantissa=14  parEnSSM=off
      settings: SourceProductName=Simulink Real-Time: Speedgoat I/O Blockset
  Encode 5 : speedgoatlib_IO682/Encode v2   parMode=Message Sequence  parLabel=101  parDataType=[2]  parResolution=[.1]  parBits=[0]  parSdi=[2]  parSsm=[0]  parCustomDataType=Raw  parDataLSB=9  parDataMSB=31  parBitPosition=[9, 31]  parScaleBNR=1  parExponent=8  parMantissa=14  parEnSSM=off
      settings: SourceProductName=Simulink Real-Time: Speedgoat I/O Blockset
  Mux : Mux
  Prepare RAW value : Subsystem
  Random number : RandomNumber  Mean=650  Variance=10  SampleTime=Ts_IO682
  Sine wave : Sin  Amplitude=10000  Bias=23000  Frequency=2*pi*0.01  SampleTime=Ts_IO682
  Out1 : Outport
  wires:
  Mux/1 -> Out1/1
  Sine wave/1 -> Encode 3/1
  Encode 2/1 -> Mux/4
  Encode 3/1 -> Mux/3
  Encode 5/1 -> Mux/2
  Random number/1 -> Encode 1/1
  Encode 1/1 -> Mux/1
  Counter Limited/1 -> Data Type Conversion/1
  Prepare RAW value/1(Out1) -> Encode 2/1
  Constant/1 -> Prepare RAW value/1(In1)
  Data Type Conversion/1 -> Encode 5/1

== system speedgoat_test_SN5659_R2021b/IO682/Encode Channel 14 ==
  Constant : Constant  Value=700.159  SampleTime=Ts_IO682
  Counter Limited : simulink/Sources/Counter Limited  uplimit=1400  tsamp=Ts_IO682
  Data Type Conversion : DataTypeConversion
  Encode 1 : speedgoatlib_IO682/Encode v2   parMode=Message Sequence  parLabel=100  parDataType=[1]  parResolution=[1024]  parBits=[10]  parSdi=[2]  parSsm=[3]  parCustomDataType=Raw  parDataLSB=9  parDataMSB=31  parBitPosition=[9, 31]  parScaleBNR=1  parExponent=8  parMantissa=14  parEnSSM=off
      settings: SourceProductName=Simulink Real-Time: Speedgoat I/O Blockset
  Encode 2 : speedgoatlib_IO682/Encode v2   parMode=Message Sequence  parLabel=101  parDataType=[2]  parResolution=[.1]  parBits=[0]  parSdi=[2]  parSsm=[0]  parCustomDataType=Raw  parDataLSB=9  parDataMSB=31  parBitPosition=[9, 31]  parScaleBNR=1  parExponent=8  parMantissa=14  parEnSSM=off
      settings: SourceProductName=Simulink Real-Time: Speedgoat I/O Blockset
  Encode 3 : speedgoatlib_IO682/Encode v2   parMode=Message Sequence  parLabel=102  parDataType=[1]  parResolution=[65536]  parBits=[16]  parSdi=[2]  parSsm=[3]  parCustomDataType=Raw  parDataLSB=9  parDataMSB=31  parBitPosition=[9, 31]  parScaleBNR=1  parExponent=8  parMantissa=14  parEnSSM=off
      settings: SourceProductName=Simulink Real-Time: Speedgoat I/O Blockset
  Encode 4 : speedgoatlib_IO682/Encode v2   parMode=Message Sequence  parLabel=103  parDataType=[0]  parResolution=[1]  parBits=[0]  parSdi=[0]  parSsm=[0]  parCustomDataType=Raw  parDataLSB=9  parDataMSB=31  parBitPosition=[9, 31]  parScaleBNR=1  parExponent=8  parMantissa=14  parEnSSM=off
      settings: SourceProductName=Simulink Real-Time: Speedgoat I/O Blockset
  Mux1 : Mux
  Prepare RAW value : Subsystem
  Random number : RandomNumber  Mean=700  Variance=10  SampleTime=Ts_IO682
  Sine wave : Sin  Amplitude=10000  Bias=24000  Frequency=2*pi*0.01  SampleTime=Ts_IO682
  Out1 : Outport
  wires:
  Encode 2/1 -> Mux1/2
  Prepare RAW value/1(Out1) -> Encode 4/1
  Encode 3/1 -> Mux1/3
  Encode 1/1 -> Mux1/1
  Constant/1 -> Prepare RAW value/1(In1)
  Sine wave/1 -> Encode 3/1
  Random number/1 -> Encode 1/1
  Mux1/1 -> Out1/1
  Counter Limited/1 -> Data Type Conversion/1
  Encode 4/1 -> Mux1/4
  Data Type Conversion/1 -> Encode 2/1

== system speedgoat_test_SN5659_R2021b/IO682/Encode Channel 15 ==
  Constant : Constant  Value=750.159  SampleTime=Ts_IO682
  Counter Limited : simulink/Sources/Counter Limited  uplimit=1500  tsamp=Ts_IO682
  Data Type Conversion : DataTypeConversion
  Encode 1 : speedgoatlib_IO682/Encode v2   parMode=Message Sequence  parLabel=100  parDataType=[1]  parResolution=[1024]  parBits=[10]  parSdi=[2]  parSsm=[3]  parCustomDataType=Raw  parDataLSB=9  parDataMSB=31  parBitPosition=[9, 31]  parScaleBNR=1  parExponent=8  parMantissa=14  parEnSSM=off
      settings: SourceProductName=Simulink Real-Time: Speedgoat I/O Blockset
  Encode 2 : speedgoatlib_IO682/Encode v2   parMode=Message Sequence  parLabel=101  parDataType=[2]  parResolution=[.1]  parBits=[0]  parSdi=[2]  parSsm=[0]  parCustomDataType=Raw  parDataLSB=9  parDataMSB=31  parBitPosition=[9, 31]  parScaleBNR=1  parExponent=8  parMantissa=14  parEnSSM=off
      settings: SourceProductName=Simulink Real-Time: Speedgoat I/O Blockset
  Encode 3 : speedgoatlib_IO682/Encode v2   parMode=Message Sequence  parLabel=102  parDataType=[1]  parResolution=[65536]  parBits=[16]  parSdi=[2]  parSsm=[3]  parCustomDataType=Raw  parDataLSB=9  parDataMSB=31  parBitPosition=[9, 31]  parScaleBNR=1  parExponent=8  parMantissa=14  parEnSSM=off
      settings: SourceProductName=Simulink Real-Time: Speedgoat I/O Blockset
  Encode 4 : speedgoatlib_IO682/Encode v2   parMode=Message Sequence  parLabel=103  parDataType=[0]  parResolution=[1]  parBits=[0]  parSdi=[0]  parSsm=[0]  parCustomDataType=Raw  parDataLSB=9  parDataMSB=31  parBitPosition=[9, 31]  parScaleBNR=1  parExponent=8  parMantissa=14  parEnSSM=off
      settings: SourceProductName=Simulink Real-Time: Speedgoat I/O Blockset
  Mux1 : Mux
  Prepare RAW value : Subsystem
  Random number : RandomNumber  Mean=750  Variance=10  SampleTime=Ts_IO682
  Sine wave : Sin  Amplitude=10000  Bias=25000  Frequency=2*pi*0.01  SampleTime=Ts_IO682
  Out1 : Outport
  wires:
  Encode 4/1 -> Mux1/4
  Mux1/1 -> Out1/1
  Counter Limited/1 -> Data Type Conversion/1
  Sine wave/1 -> Encode 3/1
  Encode 3/1 -> Mux1/3
  Encode 1/1 -> Mux1/1
  Random number/1 -> Encode 1/1
  Encode 2/1 -> Mux1/2
  Prepare RAW value/1(Out1) -> Encode 4/1
  Constant/1 -> Prepare RAW value/1(In1)
  Data Type Conversion/1 -> Encode 2/1

== system speedgoat_test_SN5659_R2021b/IO682/Encode Channel 16 ==
  Constant : Constant  Value=800.159  SampleTime=Ts_IO682
  Counter Limited : simulink/Sources/Counter Limited  uplimit=1600  tsamp=Ts_IO682
  Data Type Conversion : DataTypeConversion
  Encode 1 : speedgoatlib_IO682/Encode v2   parMode=Message Sequence  parLabel=100  parDataType=[1]  parResolution=[1024]  parBits=[10]  parSdi=[2]  parSsm=[3]  parCustomDataType=Raw  parDataLSB=9  parDataMSB=31  parBitPosition=[9, 31]  parScaleBNR=1  parExponent=8  parMantissa=14  parEnSSM=off
      settings: SourceProductName=Simulink Real-Time: Speedgoat I/O Blockset
  Encode 2 : speedgoatlib_IO682/Encode v2   parMode=Message Sequence  parLabel=101  parDataType=[2]  parResolution=[.1]  parBits=[0]  parSdi=[2]  parSsm=[0]  parCustomDataType=Raw  parDataLSB=9  parDataMSB=31  parBitPosition=[9, 31]  parScaleBNR=1  parExponent=8  parMantissa=14  parEnSSM=off
      settings: SourceProductName=Simulink Real-Time: Speedgoat I/O Blockset
  Encode 3 : speedgoatlib_IO682/Encode v2   parMode=Message Sequence  parLabel=102  parDataType=[1]  parResolution=[65536]  parBits=[16]  parSdi=[2]  parSsm=[3]  parCustomDataType=Raw  parDataLSB=9  parDataMSB=31  parBitPosition=[9, 31]  parScaleBNR=1  parExponent=8  parMantissa=14  parEnSSM=off
      settings: SourceProductName=Simulink Real-Time: Speedgoat I/O Blockset
  Encode 4 : speedgoatlib_IO682/Encode v2   parMode=Message Sequence  parLabel=103  parDataType=[0]  parResolution=[1]  parBits=[0]  parSdi=[0]  parSsm=[0]  parCustomDataType=Raw  parDataLSB=9  parDataMSB=31  parBitPosition=[9, 31]  parScaleBNR=1  parExponent=8  parMantissa=14  parEnSSM=off
      settings: SourceProductName=Simulink Real-Time: Speedgoat I/O Blockset
  Mux1 : Mux
  Prepare RAW value : Subsystem
  Random number : RandomNumber  Mean=800  Variance=10  SampleTime=Ts_IO682
  Sine wave : Sin  Amplitude=10000  Bias=26000  Frequency=2*pi*0.01  SampleTime=Ts_IO682
  Out1 : Outport
  wires:
  Encode 4/1 -> Mux1/4
  Mux1/1 -> Out1/1
  Counter Limited/1 -> Data Type Conversion/1
  Sine wave/1 -> Encode 3/1
  Encode 3/1 -> Mux1/3
  Encode 1/1 -> Mux1/1
  Random number/1 -> Encode 1/1
  Encode 2/1 -> Mux1/2
  Prepare RAW value/1(Out1) -> Encode 4/1
  Constant/1 -> Prepare RAW value/1(In1)
  Data Type Conversion/1 -> Encode 2/1

== system speedgoat_test_SN5659_R2021b/IO682/Encode Channel 2 ==
  Constant : Constant  Value=100.159  SampleTime=Ts_IO682
  Counter Limited : simulink/Sources/Counter Limited  uplimit=200  tsamp=Ts_IO682
  Data Type Conversion : DataTypeConversion
  Encode 1 : speedgoatlib_IO682/Encode v2   parMode=Message Sequence  parLabel=100  parDataType=[1]  parResolution=[1024]  parBits=[10]  parSdi=[2]  parSsm=[3]  parCustomDataType=Raw  parDataLSB=9  parDataMSB=31  parBitPosition=[9, 31]  parScaleBNR=1  parExponent=8  parMantissa=14  parEnSSM=off
      settings: SourceProductName=Simulink Real-Time: Speedgoat I/O Blockset
  Encode 2 : speedgoatlib_IO682/Encode v2   parMode=Message Sequence  parLabel=101  parDataType=[2]  parResolution=[.1]  parBits=[0]  parSdi=[2]  parSsm=[0]  parCustomDataType=Raw  parDataLSB=9  parDataMSB=31  parBitPosition=[9, 31]  parScaleBNR=1  parExponent=8  parMantissa=14  parEnSSM=off
      settings: SourceProductName=Simulink Real-Time: Speedgoat I/O Blockset
  Encode 3 : speedgoatlib_IO682/Encode v2   parMode=Message Sequence  parLabel=102  parDataType=[1]  parResolution=[65536]  parBits=[16]  parSdi=[2]  parSsm=[3]  parCustomDataType=Raw  parDataLSB=9  parDataMSB=31  parBitPosition=[9, 31]  parScaleBNR=1  parExponent=8  parMantissa=14  parEnSSM=off
      settings: SourceProductName=Simulink Real-Time: Speedgoat I/O Blockset
  Encode 4 : speedgoatlib_IO682/Encode v2   parMode=Message Sequence  parLabel=103  parDataType=[0]  parResolution=[1]  parBits=[0]  parSdi=[0]  parSsm=[0]  parCustomDataType=Raw  parDataLSB=9  parDataMSB=31  parBitPosition=[9, 31]  parScaleBNR=1  parExponent=8  parMantissa=14  parEnSSM=off
      settings: SourceProductName=Simulink Real-Time: Speedgoat I/O Blockset
  Mux1 : Mux
  Prepare RAW value : Subsystem
  Random number : RandomNumber  Mean=100  Variance=10  SampleTime=Ts_IO682
  Sine wave : Sin  Amplitude=10000  Bias=12000  Frequency=2*pi*0.01  SampleTime=Ts_IO682
  Out1 : Outport
  wires:
  Encode 2/1 -> Mux1/2
  Prepare RAW value/1(Out1) -> Encode 4/1
  Encode 3/1 -> Mux1/3
  Encode 1/1 -> Mux1/1
  Constant/1 -> Prepare RAW value/1(In1)
  Sine wave/1 -> Encode 3/1
  Random number/1 -> Encode 1/1
  Mux1/1 -> Out1/1
  Counter Limited/1 -> Data Type Conversion/1
  Encode 4/1 -> Mux1/4
  Data Type Conversion/1 -> Encode 2/1
